simulink model "part3"  (R2015a)
settings: Solver=ode3  StartTime=0.0  StopTime=100  FixedStep=0.1  RelTol=1e-8
values from neighbouring files (symbols this model uses):
  g = 9.81    [env.m]
  K = [2*g; 1]    [env.m]
  l = 10    [env.m]
  ue = 0    [env.m]
  xe = [0; 0]    [env.m]
libraries: simulink x1
settings Model: Creator=vdrouinv  LastModifiedBy=vdrouinv

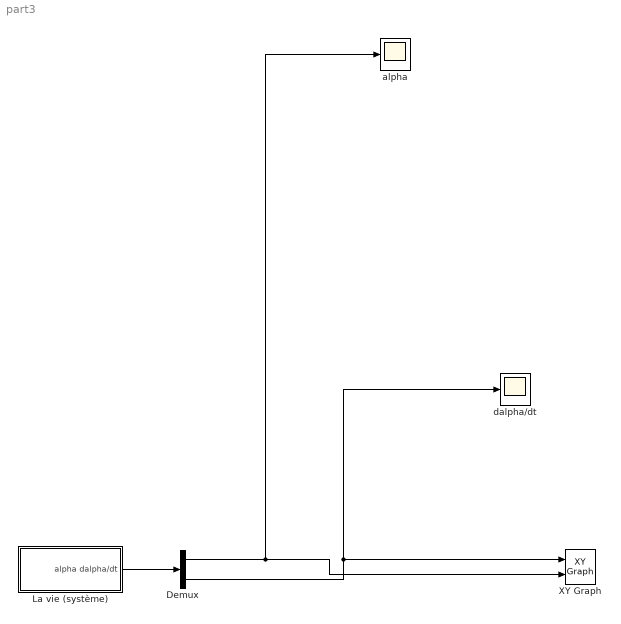
== system part3 ==
  Demux : Demux  Outputs=2
  La vie (système) : Subsystem
  XY Graph : simulink/Sinks/XY Graph  xmin=-10  xmax=10  ymin=-10  ymax=10  st=-1
  alpha : Scope
  dalpha/dt : Scope
  wires:
  La vie (système)/1(alpha dalpha/dt) -> Demux/1
  Demux/1 -> XY Graph/2, alpha/1
  Demux/2 -> dalpha/dt/1, XY Graph/1

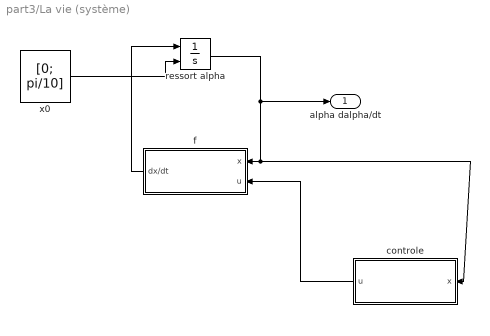
== system part3/La vie (système) ==
  controle : Subsystem  TreatAsAtomicUnit=on
  f : Subsystem  TreatAsAtomicUnit=on
  ressort alpha : Integrator  InitialConditionSource=external
  x0 : Constant  Value=[0; pi/10]
  alpha dalpha/dt : Outport
  wires:
  x0/1 -> ressort alpha/2
  f/1(dx/dt) -> ressort alpha/1
  ressort alpha/1 -> controle/1(x), f/1(x), alpha dalpha/dt/1
  controle/1(u) -> f/2(u)

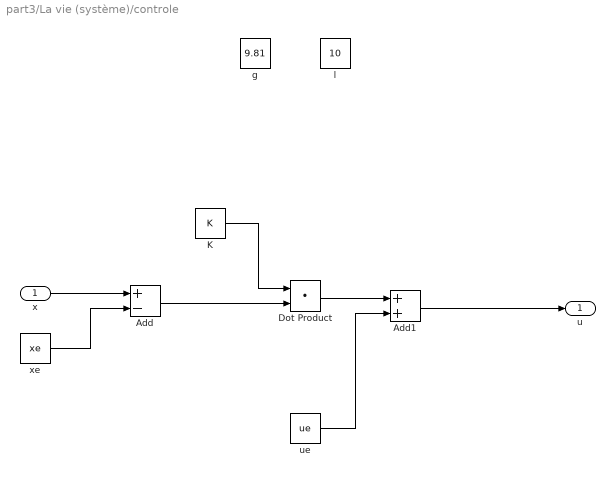
== system part3/La vie (système)/controle ==
  x : Inport
  Add : Sum  Inputs=+-
  Add1 : Sum
  Dot Product : DotProduct  InputSameDT=on  OutDataTypeStr=Inherit: Inherit via internal rule
  K : Constant  Value=K
  g : Constant  Value=9.81
  l : Constant  Value=10
  ue : Constant  Value=ue
  xe : Constant  Value=xe
  u : Outport
  wires:
  x/1 -> Add/1
  xe/1 -> Add/2
  Add/1 -> Dot Product/2
  K/1 -> Dot Product/1
  Dot Product/1 -> Add1/1
  ue/1 -> Add1/2
  Add1/1 -> u/1

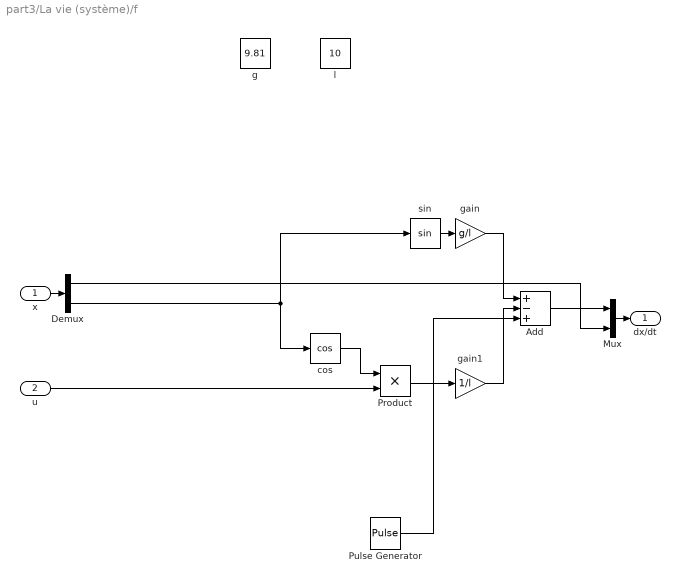
== system part3/La vie (système)/f ==
  x : Inport
  u : Inport  Port=2
  " gain" : Gain  Gain=g/l
  " gain1" : Gain  Gain=1/l
  Add : Sum  Inputs=+-+
  Demux : Demux  Outputs=2
  Mux : Mux  Inputs=2
  Product : Product
  Pulse Generator : DiscretePulseGenerator  PulseType=Time based  Amplitude=10  Period=10
  cos : Trigonometry  Operator=cos
  g : Constant  Value=9.81
  l : Constant  Value=10
  sin : Trigonometry
  dx/dt : Outport
  wires:
  Demux/2 -> cos/1, sin/1
  x/1 -> Demux/1
  sin/1 -> " gain"/1
  Mux/1 -> dx/dt/1
  u/1 -> Product/2
  cos/1 -> Product/1
  Product/1 -> " gain1"/1
  " gain1"/1 -> Add/2
  " gain"/1 -> Add/1
  Add/1 -> Mux/1
  Demux/1 -> Mux/2
  Pulse Generator/1 -> Add/3
